simulink model "Hopf_oscillator_4legs"  (R2021b)
settings: Solver=ode23  StartTime=0.0  StopTime=10  RelTol=1e-6
undefined symbols (not defined in the file): A, alpha, epsilon, f, init_state, k, phi_vec, tau
settings Model: Creator=kaiget  LastModifiedBy=kaiget

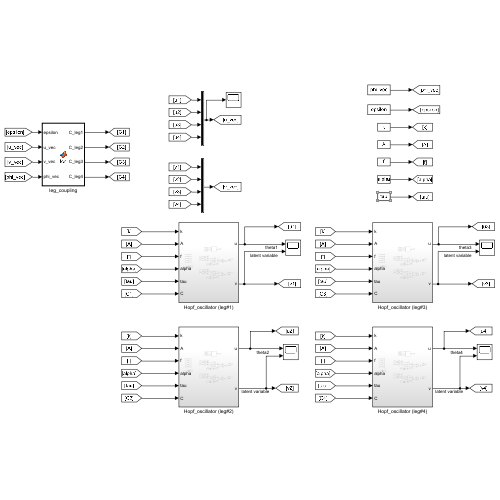
[thumbnail: Simulink's stored preview of the top-level diagram]
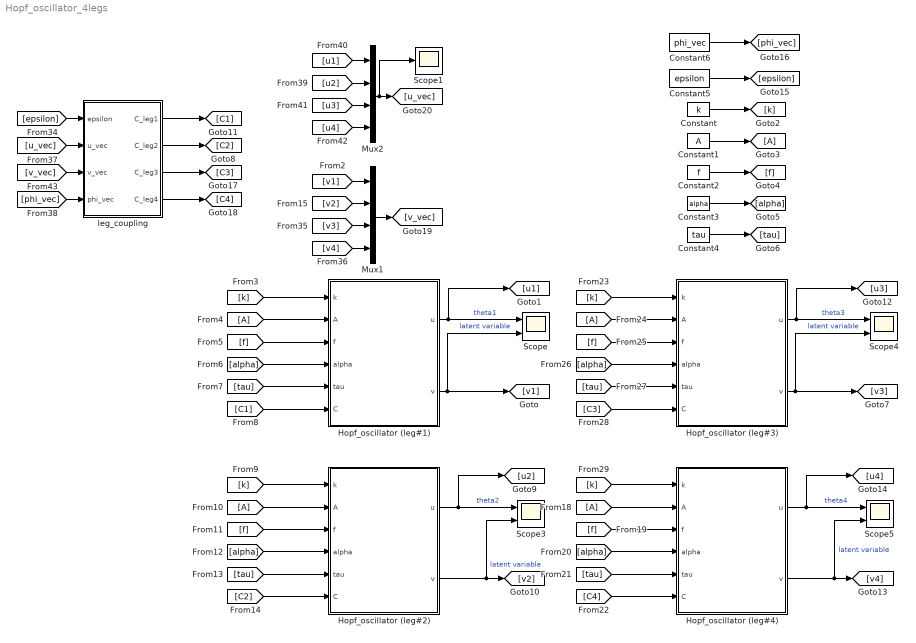
== system Hopf_oscillator_4legs ==
  Constant : Constant  Value=k
  Constant1 : Constant  Value=A
  Constant2 : Constant  Value=f
  Constant3 : Constant  Value=alpha
  Constant4 : Constant  Value=tau
  Constant5 : Constant  Value=epsilon
  Constant6 : Constant  Value=phi_vec
  Hopf_oscillator (leg#1) : Subsystem
  Hopf_oscillator (leg#2) : Subsystem
  Hopf_oscillator (leg#3) : Subsystem
  Hopf_oscillator (leg#4) : Subsystem
  Mux1 : Mux
  Mux2 : Mux
  Scope{,3..5} (4 alike) : Scope  NumInputPorts=2
  Scope1 : Scope
  leg_coupling : MATLAB Function  TreatAsAtomicUnit=on
  wires:
  [k] -> Hopf_oscillator (leg#1)/1(k)
  [A] -> Hopf_oscillator (leg#1)/2(A)
  [f] -> Hopf_oscillator (leg#1)/3(f)
  [alpha] -> Hopf_oscillator (leg#1)/4(alpha)
  [tau] -> Hopf_oscillator (leg#1)/5(tau)
  [C1] -> Hopf_oscillator (leg#1)/6(C)
  Hopf_oscillator (leg#1)/1(u) -> [u1], Scope/1  "theta1"
  Hopf_oscillator (leg#1)/2(v) -> [v1], Scope/2  "latent variable"
  [v1] -> Mux1/1
  Hopf_oscillator (leg#2)/2(v) -> [v2], Scope3/2  "latent variable"
  Constant/1 -> [k]
  Constant1/1 -> [A]
  Constant2/1 -> [f]
  Constant3/1 -> [alpha]
  Constant4/1 -> [tau]
  [k] -> Hopf_oscillator (leg#2)/1(k)
  [A] -> Hopf_oscillator (leg#2)/2(A)
  [f] -> Hopf_oscillator (leg#2)/3(f)
  [alpha] -> Hopf_oscillator (leg#2)/4(alpha)
  [tau] -> Hopf_oscillator (leg#2)/5(tau)
  [C2] -> Hopf_oscillator (leg#2)/6(C)
  Hopf_oscillator (leg#2)/1(u) -> [u2], Scope3/1  "theta2"
  [v2] -> Mux1/2
  Hopf_oscillator (leg#3)/1(u) -> [u3], Scope4/1  "theta3"
  [alpha] -> Hopf_oscillator (leg#4)/4(alpha)
  [f] -> Hopf_oscillator (leg#4)/3(f)
  Hopf_oscillator (leg#4)/1(u) -> [u4], Scope5/1  "theta4"
  [C4] -> Hopf_oscillator (leg#4)/6(C)
  [k] -> Hopf_oscillator (leg#4)/1(k)
  [tau] -> Hopf_oscillator (leg#3)/5(tau)
  [A] -> Hopf_oscillator (leg#4)/2(A)
  [f] -> Hopf_oscillator (leg#3)/3(f)
  [alpha] -> Hopf_oscillator (leg#3)/4(alpha)
  Hopf_oscillator (leg#4)/2(v) -> [v4], Scope5/2  "latent variable"
  [tau] -> Hopf_oscillator (leg#4)/5(tau)
  Hopf_oscillator (leg#3)/2(v) -> [v3], Scope4/2  "latent variable"
  [A] -> Hopf_oscillator (leg#3)/2(A)
  [C3] -> Hopf_oscillator (leg#3)/6(C)
  [k] -> Hopf_oscillator (leg#3)/1(k)
  Constant5/1 -> [epsilon]
  leg_coupling/1(C_leg1) -> [C1]
  leg_coupling/2(C_leg2) -> [C2]
  leg_coupling/3(C_leg3) -> [C3]
  leg_coupling/4(C_leg4) -> [C4]
  [epsilon] -> leg_coupling/1(epsilon)
  [v3] -> Mux1/3
  [v4] -> Mux1/4
  Mux1/1 -> [v_vec]
  [u_vec] -> leg_coupling/2(u_vec)
  [phi_vec] -> leg_coupling/4(phi_vec)
  Mux2/1 -> Scope1/1, [u_vec]
  [u3] -> Mux2/3
  [u4] -> Mux2/4
  [u1] -> Mux2/1
  [u2] -> Mux2/2
  [v_vec] -> leg_coupling/3(v_vec)
  Constant6/1 -> [phi_vec]

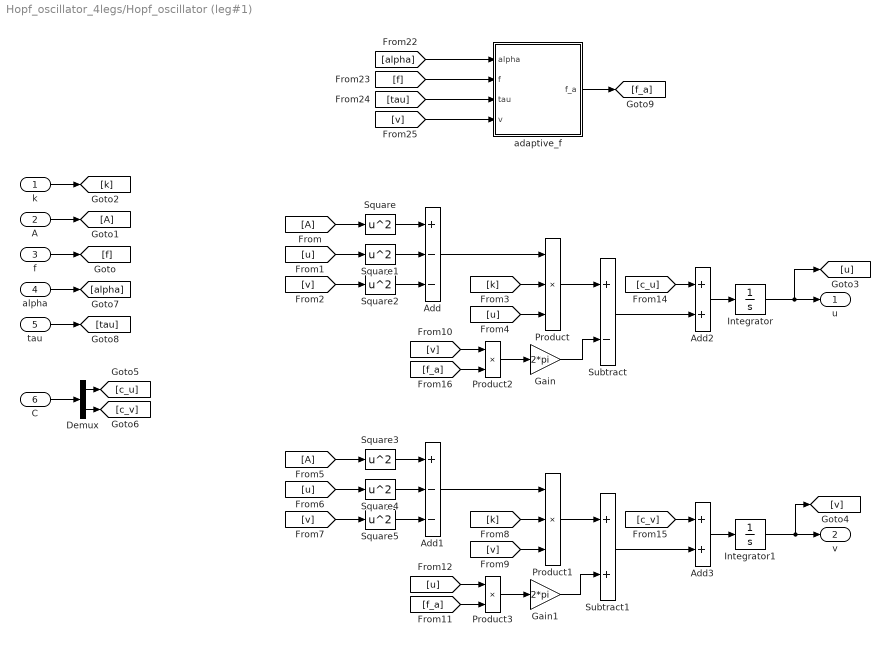
== system Hopf_oscillator_4legs/Hopf_oscillator (leg#1) ==
  k : Inport
  A : Inport  Port=2
  f : Inport  Port=3
  alpha : Inport  Port=4
  tau : Inport  Port=5
  C : Inport  Port=6
  Add : Sum  Inputs=+--
  Add1 : Sum  Inputs=+--
  Add2 : Sum
  Add3 : Sum
  Demux : Demux  Outputs=2
  Gain : Gain  Gain=2*pi
  Gain1 : Gain  Gain=2*pi
  Integrator : Integrator  InitialCondition=init_state(1)
  Integrator1 : Integrator  InitialCondition=init_state(2)
  Product : Product  Inputs=3
  Product1 : Product  Inputs=3
  Product2 : Product
  Product3 : Product
  Square{,1..5} (6 alike) : Math  Operator=square  SaturateOnIntegerOverflow=on
  Subtract : Sum  Inputs=+-
  Subtract1 : Sum
  adaptive_f : MATLAB Function  TreatAsAtomicUnit=on
  u : Outport
  v : Outport  Port=2
  wires:
  Integrator/1 -> [u], u/1
  f/1 -> [f]
  A/1 -> [A]
  k/1 -> [k]
  Integrator1/1 -> [v], v/1
  [A] -> Square/1
  [u] -> Square1/1
  [v] -> Square2/1
  Square2/1 -> Add/3
  Square1/1 -> Add/2
  Square/1 -> Add/1
  Add/1 -> Product/1
  [k] -> Product/2
  [u] -> Product/3
  Product/1 -> Subtract/1
  Square3/1 -> Add1/1
  Square4/1 -> Add1/2
  Square5/1 -> Add1/3
  [v] -> Product1/3
  Product1/1 -> Subtract1/1
  [v] -> Square5/1
  [A] -> Square3/1
  [u] -> Square4/1
  Add1/1 -> Product1/1
  [k] -> Product1/2
  [v] -> Product2/1
  [f_a] -> Product2/2
  Product2/1 -> Gain/1
  Gain/1 -> Subtract/2
  [u] -> Product3/1
  Product3/1 -> Gain1/1
  [f_a] -> Product3/2
  Gain1/1 -> Subtract1/2
  Subtract/1 -> Add2/2
  C/1 -> Demux/1
  Demux/1 -> [c_u]
  Demux/2 -> [c_v]
  [c_u] -> Add2/1
  Add2/1 -> Integrator/1
  Subtract1/1 -> Add3/2
  [c_v] -> Add3/1
  Add3/1 -> Integrator1/1
  alpha/1 -> [alpha]
  tau/1 -> [tau]
  [alpha] -> adaptive_f/1(alpha)
  [f] -> adaptive_f/2(f)
  [tau] -> adaptive_f/3(tau)
  [v] -> adaptive_f/4(v)
  adaptive_f/1(f_a) -> [f_a]

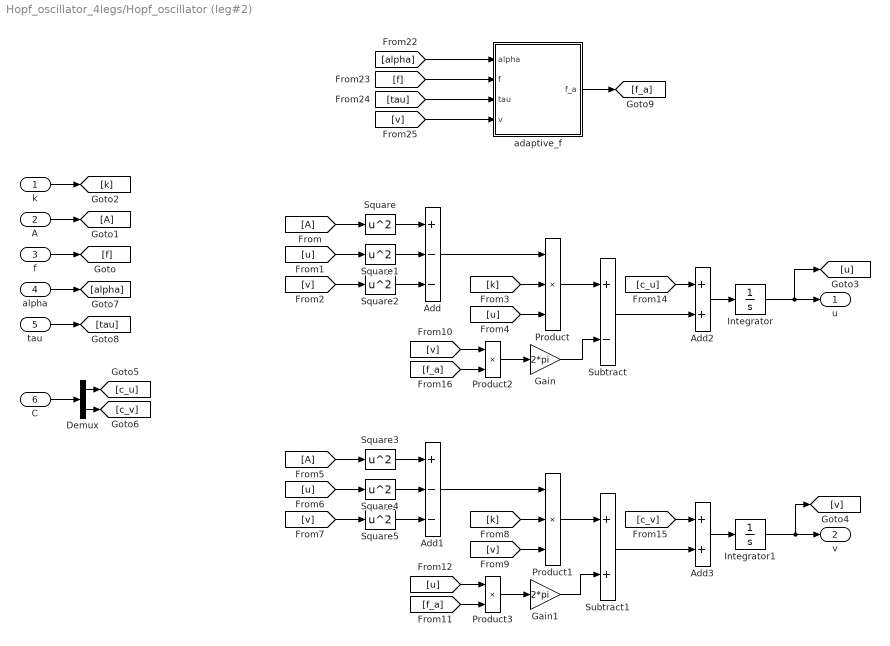
== system Hopf_oscillator_4legs/Hopf_oscillator (leg#2) ==
  k : Inport
  A : Inport  Port=2
  f : Inport  Port=3
  alpha : Inport  Port=4
  tau : Inport  Port=5
  C : Inport  Port=6
  Add : Sum  Inputs=+--
  Add1 : Sum  Inputs=+--
  Add2 : Sum
  Add3 : Sum
  Demux : Demux  Outputs=2
  Gain : Gain  Gain=2*pi
  Gain1 : Gain  Gain=2*pi
  Integrator : Integrator  InitialCondition=init_state(3)
  Integrator1 : Integrator  InitialCondition=init_state(4)
  Product : Product  Inputs=3
  Product1 : Product  Inputs=3
  Product2 : Product
  Product3 : Product
  Square{,1..5} (6 alike) : Math  Operator=square  SaturateOnIntegerOverflow=on
  Subtract : Sum  Inputs=+-
  Subtract1 : Sum
  adaptive_f : MATLAB Function  TreatAsAtomicUnit=on
  u : Outport
  v : Outport  Port=2
  wires:
  Integrator/1 -> [u], u/1
  f/1 -> [f]
  A/1 -> [A]
  k/1 -> [k]
  Integrator1/1 -> [v], v/1
  [A] -> Square/1
  [u] -> Square1/1
  [v] -> Square2/1
  Square2/1 -> Add/3
  Square1/1 -> Add/2
  Square/1 -> Add/1
  Add/1 -> Product/1
  [k] -> Product/2
  [u] -> Product/3
  Product/1 -> Subtract/1
  Square3/1 -> Add1/1
  Square4/1 -> Add1/2
  Square5/1 -> Add1/3
  [v] -> Product1/3
  Product1/1 -> Subtract1/1
  [v] -> Square5/1
  [A] -> Square3/1
  [u] -> Square4/1
  Add1/1 -> Product1/1
  [k] -> Product1/2
  [v] -> Product2/1
  [f_a] -> Product2/2
  Product2/1 -> Gain/1
  Gain/1 -> Subtract/2
  [u] -> Product3/1
  Product3/1 -> Gain1/1
  [f_a] -> Product3/2
  Gain1/1 -> Subtract1/2
  Subtract/1 -> Add2/2
  C/1 -> Demux/1
  Demux/1 -> [c_u]
  Demux/2 -> [c_v]
  [c_u] -> Add2/1
  Add2/1 -> Integrator/1
  Subtract1/1 -> Add3/2
  [c_v] -> Add3/1
  Add3/1 -> Integrator1/1
  alpha/1 -> [alpha]
  tau/1 -> [tau]
  [alpha] -> adaptive_f/1(alpha)
  [f] -> adaptive_f/2(f)
  [tau] -> adaptive_f/3(tau)
  [v] -> adaptive_f/4(v)
  adaptive_f/1(f_a) -> [f_a]

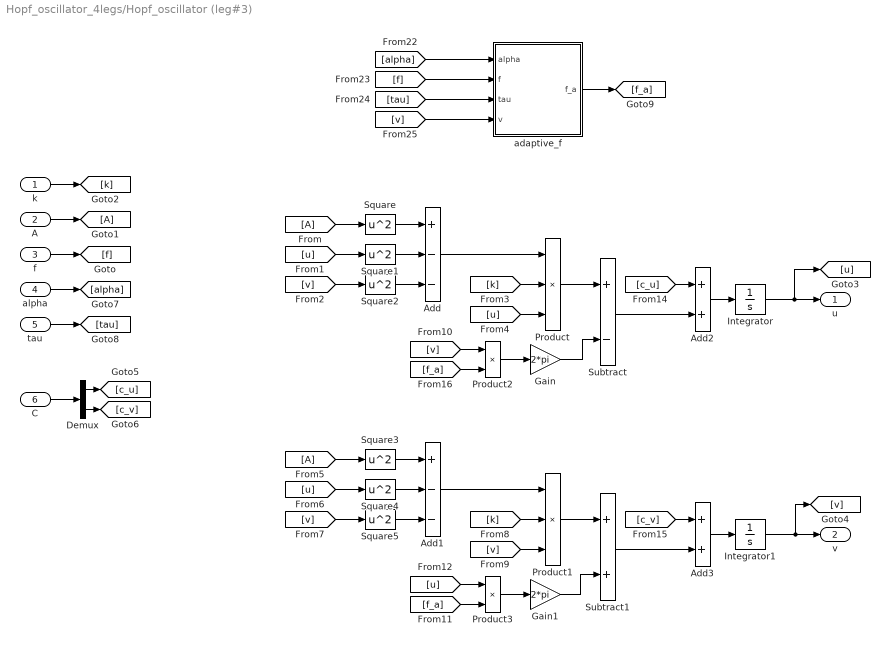
== system Hopf_oscillator_4legs/Hopf_oscillator (leg#3) ==
  k : Inport
  A : Inport  Port=2
  f : Inport  Port=3
  alpha : Inport  Port=4
  tau : Inport  Port=5
  C : Inport  Port=6
  Add : Sum  Inputs=+--
  Add1 : Sum  Inputs=+--
  Add2 : Sum
  Add3 : Sum
  Demux : Demux  Outputs=2
  Gain : Gain  Gain=2*pi
  Gain1 : Gain  Gain=2*pi
  Integrator : Integrator  InitialCondition=init_state(5)
  Integrator1 : Integrator  InitialCondition=init_state(6)
  Product : Product  Inputs=3
  Product1 : Product  Inputs=3
  Product2 : Product
  Product3 : Product
  Square{,1..5} (6 alike) : Math  Operator=square  SaturateOnIntegerOverflow=on
  Subtract : Sum  Inputs=+-
  Subtract1 : Sum
  adaptive_f : MATLAB Function  TreatAsAtomicUnit=on
  u : Outport
  v : Outport  Port=2
  wires:
  Integrator/1 -> [u], u/1
  f/1 -> [f]
  A/1 -> [A]
  k/1 -> [k]
  Integrator1/1 -> [v], v/1
  [A] -> Square/1
  [u] -> Square1/1
  [v] -> Square2/1
  Square2/1 -> Add/3
  Square1/1 -> Add/2
  Square/1 -> Add/1
  Add/1 -> Product/1
  [k] -> Product/2
  [u] -> Product/3
  Product/1 -> Subtract/1
  Square3/1 -> Add1/1
  Square4/1 -> Add1/2
  Square5/1 -> Add1/3
  [v] -> Product1/3
  Product1/1 -> Subtract1/1
  [v] -> Square5/1
  [A] -> Square3/1
  [u] -> Square4/1
  Add1/1 -> Product1/1
  [k] -> Product1/2
  [v] -> Product2/1
  [f_a] -> Product2/2
  Product2/1 -> Gain/1
  Gain/1 -> Subtract/2
  [u] -> Product3/1
  Product3/1 -> Gain1/1
  [f_a] -> Product3/2
  Gain1/1 -> Subtract1/2
  Subtract/1 -> Add2/2
  C/1 -> Demux/1
  Demux/1 -> [c_u]
  Demux/2 -> [c_v]
  [c_u] -> Add2/1
  Add2/1 -> Integrator/1
  Subtract1/1 -> Add3/2
  [c_v] -> Add3/1
  Add3/1 -> Integrator1/1
  alpha/1 -> [alpha]
  tau/1 -> [tau]
  [alpha] -> adaptive_f/1(alpha)
  [f] -> adaptive_f/2(f)
  [tau] -> adaptive_f/3(tau)
  [v] -> adaptive_f/4(v)
  adaptive_f/1(f_a) -> [f_a]

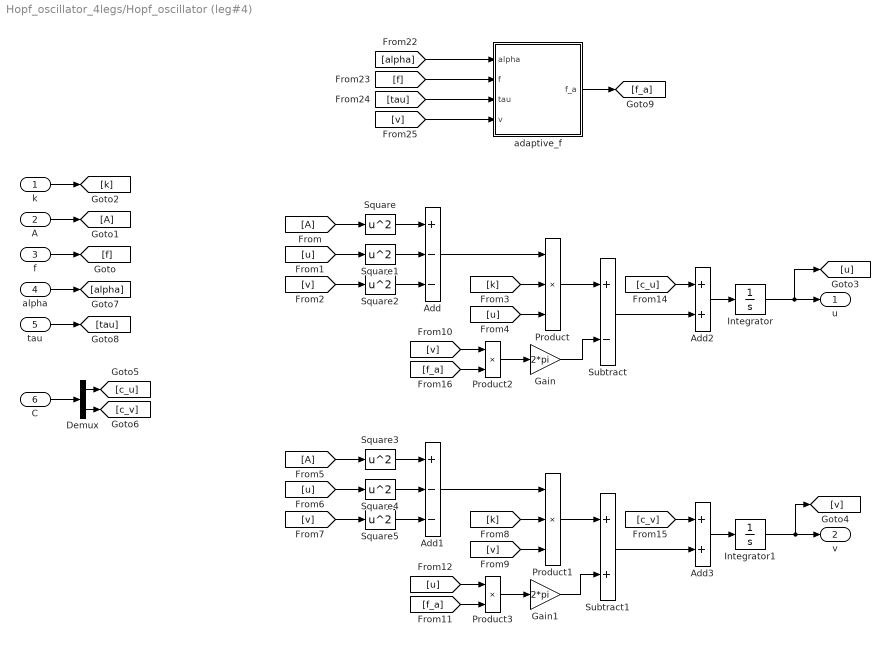
== system Hopf_oscillator_4legs/Hopf_oscillator (leg#4) ==
  k : Inport
  A : Inport  Port=2
  f : Inport  Port=3
  alpha : Inport  Port=4
  tau : Inport  Port=5
  C : Inport  Port=6
  Add : Sum  Inputs=+--
  Add1 : Sum  Inputs=+--
  Add2 : Sum
  Add3 : Sum
  Demux : Demux  Outputs=2
  Gain : Gain  Gain=2*pi
  Gain1 : Gain  Gain=2*pi
  Integrator : Integrator  InitialCondition=init_state(7)
  Integrator1 : Integrator  InitialCondition=init_state(8)
  Product : Product  Inputs=3
  Product1 : Product  Inputs=3
  Product2 : Product
  Product3 : Product
  Square{,1..5} (6 alike) : Math  Operator=square  SaturateOnIntegerOverflow=on
  Subtract : Sum  Inputs=+-
  Subtract1 : Sum
  adaptive_f : MATLAB Function  TreatAsAtomicUnit=on
  u : Outport
  v : Outport  Port=2
  wires:
  Integrator/1 -> [u], u/1
  f/1 -> [f]
  A/1 -> [A]
  k/1 -> [k]
  Integrator1/1 -> [v], v/1
  [A] -> Square/1
  [u] -> Square1/1
  [v] -> Square2/1
  Square2/1 -> Add/3
  Square1/1 -> Add/2
  Square/1 -> Add/1
  Add/1 -> Product/1
  [k] -> Product/2
  [u] -> Product/3
  Product/1 -> Subtract/1
  Square3/1 -> Add1/1
  Square4/1 -> Add1/2
  Square5/1 -> Add1/3
  [v] -> Product1/3
  Product1/1 -> Subtract1/1
  [v] -> Square5/1
  [A] -> Square3/1
  [u] -> Square4/1
  Add1/1 -> Product1/1
  [k] -> Product1/2
  [v] -> Product2/1
  [f_a] -> Product2/2
  Product2/1 -> Gain/1
  Gain/1 -> Subtract/2
  [u] -> Product3/1
  Product3/1 -> Gain1/1
  [f_a] -> Product3/2
  Gain1/1 -> Subtract1/2
  Subtract/1 -> Add2/2
  C/1 -> Demux/1
  Demux/1 -> [c_u]
  Demux/2 -> [c_v]
  [c_u] -> Add2/1
  Add2/1 -> Integrator/1
  Subtract1/1 -> Add3/2
  [c_v] -> Add3/1
  Add3/1 -> Integrator1/1
  alpha/1 -> [alpha]
  tau/1 -> [tau]
  [alpha] -> adaptive_f/1(alpha)
  [f] -> adaptive_f/2(f)
  [tau] -> adaptive_f/3(tau)
  [v] -> adaptive_f/4(v)
  adaptive_f/1(f_a) -> [f_a]

== matlab function Hopf_oscillator_4legs/Hopf_oscillator (leg#2)/adaptive_f ==
  data: alpha input; f_a output; f input; tau input; v input
 % calculate the adaptive frequency f through (4) in 
 % 'Design and Locomotion Control of a Biomimetic Underwater Vehicle ... '
function f_a = adaptive_f(alpha, f, tau, v)
    f1 = f/2/alpha;
    f2 = (2*alpha - 1)*f/(2*alpha*(1 - alpha)*(1 + exp(-tau*v)));
    f_a = f1 + f2;

== matlab function Hopf_oscillator_4legs/Hopf_oscillator (leg#1)/adaptive_f ==
  data: alpha input; f_a output; f input; tau input; v input
 % calculate the adaptive frequency f through (4) in 
 % 'Design and Locomotion Control of a Biomimetic Underwater Vehicle ... '
function f_a = adaptive_f(alpha, f, tau, v)
    f1 = f/2/alpha;
    f2 = (2*alpha - 1)*f/(2*alpha*(1 - alpha)*(1 + exp(-tau*v)));
    f_a = f1 + f2;

== matlab function Hopf_oscillator_4legs/Hopf_oscillator (leg#3)/adaptive_f ==
  data: alpha input; f_a output; f input; tau input; v input
 % calculate the adaptive frequency f through (4) in 
 % 'Design and Locomotion Control of a Biomimetic Underwater Vehicle ... '
function f_a = adaptive_f(alpha, f, tau, v)
    f1 = f/2/alpha;
    f2 = (2*alpha - 1)*f/(2*alpha*(1 - alpha)*(1 + exp(-tau*v)));
    f_a = f1 + f2;

== matlab function Hopf_oscillator_4legs/Hopf_oscillator (leg#4)/adaptive_f ==
  data: alpha input; f_a output; f input; tau input; v input
 % calculate the adaptive frequency f through (4) in 
 % 'Design and Locomotion Control of a Biomimetic Underwater Vehicle ... '
function f_a = adaptive_f(alpha, f, tau, v)
    f1 = f/2/alpha;
    f2 = (2*alpha - 1)*f/(2*alpha*(1 - alpha)*(1 + exp(-tau*v)));
    f_a = f1 + f2;

== matlab function Hopf_oscillator_4legs/leg_coupling ==
  data: epsilon input; u_vec input; C_leg1 output size=2; v_vec input; phi_vec input; C_leg2 output size=2; C_leg3 output size=2; C_leg4 output size=2
% epsilon: 1X1
% u_vec: 4X1
% v_vec: 4X1
% phi_vec: 4X1
% C_leg1-4 : 2X1
function [C_leg1, C_leg2, C_leg3, C_leg4] = fcn(epsilon, u_vec, v_vec, phi_vec)
    C1 = 0;
    % first leg
    C21 = epsilon*(-u_vec(4)*sin(phi_vec(4)) + v_vec(4)*cos(phi_vec(4)) - ...
                   -u_vec(1)*sin(phi_vec(1)) + v_vec(2)*cos(phi_vec(1)));
    C22 = epsilon*(-u_vec(1)*sin(phi_vec(1)) + v_vec(1)*cos(phi_vec(1)) - ...
                   -u_vec(2)*sin(phi_vec(2)) + v_vec(3)*cos(phi_vec(2)));
    C23 = epsilon*(-u_vec(2)*sin(phi_vec(2)) + v_vec(2)*cos(phi_vec(2)) - ...
                   -u_vec(3)*sin(phi_vec(3)) + v_vec(4)*cos(phi_vec(3)));
    C24 = epsilon*(-u_vec(3)*sin(phi_vec(3)) + v_vec(3)*cos(phi_vec(3)) - ...
                   -u_vec(4)*sin(phi_vec(4)) + v_vec(1)*cos(phi_vec(4)));
    
    C_leg1 = [C1; C21];
    C_leg2 = [C1; C22];
    C_leg3 = [C1; C23];
    C_leg4 = [C1; C24];
